simulink model "power_quality_digitalflickermeter"  (R2023a)
settings: Solver=VariableStepAuto  StartTime=0.0  StopTime=650  RelTol=1e-3
libraries: spsDigitalFlickermeterLib x1
settings Model: Creator=kchong  LastModifiedBy=kchong

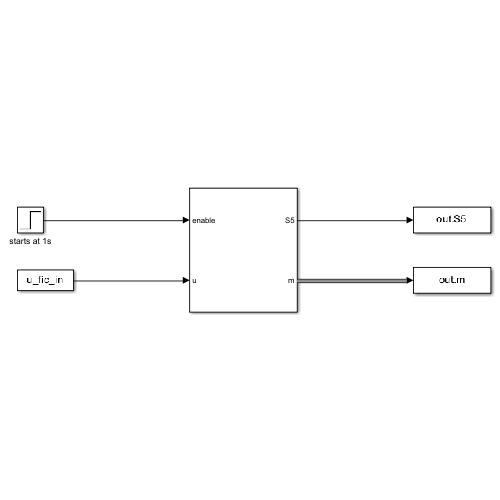
[thumbnail: Simulink's stored preview of the top-level diagram]
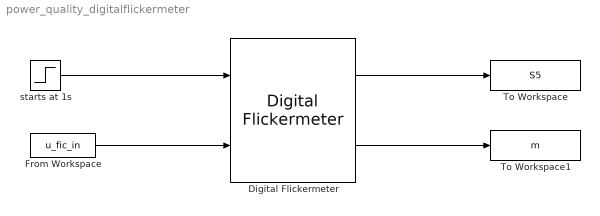
== system power_quality_digitalflickermeter ==
  Digital Flickermeter : spsDigitalFlickermeterLib/Digital Flickermeter  N_freq=60 Hz  V_R=12e3/sqrt(3)  Lim_1=5.0  Lim_5=1000  Ts=0.00002  Gain=1.24e6  type_volt=120 Vrms/60 Hz  type_fluc=Sinusoidal  Parameter12=on  fmx=8.8 Hz  dVx=0  test_mode=off
      settings: LibrarySourceBlock=|
      | sps_lib/Sensors and Measurements/Digital
      | Flickermeter
  From Workspace : FromWorkspace  VariableName=u_fic_in
  To Workspace : ToWorkspace  VariableName=S5  SaveFormat=Structure With Time  SampleTime=-1
  To Workspace1 : ToWorkspace  VariableName=m  SaveFormat=Timeseries  SampleTime=-1
  starts at 1s : Step  SampleTime=0
  wires:
  starts at 1s/1 -> Digital Flickermeter/1
  From Workspace/1 -> Digital Flickermeter/2
  Digital Flickermeter/2 -> To Workspace1/1
  Digital Flickermeter/1 -> To Workspace/1
